simulink model "closed_pi_VS"  (R2015b)
settings: Solver=ode15s  StartTime=0.0  StopTime=16000  MaxStep=10  RelTol=1e-3
values from neighbouring files (symbols this model uses):
  alfa = 3.0    (= 3)    [project_162.m]
  den_VS = [tau_i 0]    [project_162.m]
  M1 = 6000    [project_162.m]
  M10 = 6000    [project_162.m]
  M2 = 50    [project_162.m]
  M3 = 50    [project_162.m]
  M4 = 50    [project_162.m]
  M5 = 50    [project_162.m]
  M6 = 50    [project_162.m]
  M7 = 50    [project_162.m]
  M8 = 50    [project_162.m]
  M9 = 50    [project_162.m]
  num_VS = [kc_VS*tau_i kc_VS]    [project_162.m]
  VS_final = 0    [project_162.m]
  VS_steptime = 0    [project_162.m]
settings Model: Creator=chris  LastModifiedBy=chris
settings DataIOCC: SaveFormat=Array  SignalLoggingSaveFormat=ModelDataLogs
settings OptimizationCC: InitFltsAndDblsToZero=on
settings DebuggingCC: SaveWithParameterizedLinksMsg=none  UnderspecifiedInitializationDetection=Classic  MergeDetectMultiDrivingBlocksExec=none  SignalResolutionControl=TryResolveAllWithWarning  SolverPrmCheckMsg=warning  MultiTaskDSMMsg=warning  MultiTaskCondExecSysMsg=none  FcnCallInpInsideContextMsg=UseLocalSettings
settings HardwareCC: ProdBitPerPointer=32  ProdLargestAtomicFloat=None  ProdIntDivRoundTo=Undefined  ProdEndianess=Unspecified  ProdWordSize=32  ProdHWDeviceType=32-bit Generic
settings GRTTargetCC: TargetFcnLib=ansi_tfl_tmw.mat  CombineOutputUpdateFcns=off  GRTInterface=on
settings ConfigComp: CovModelRefEnable=Off

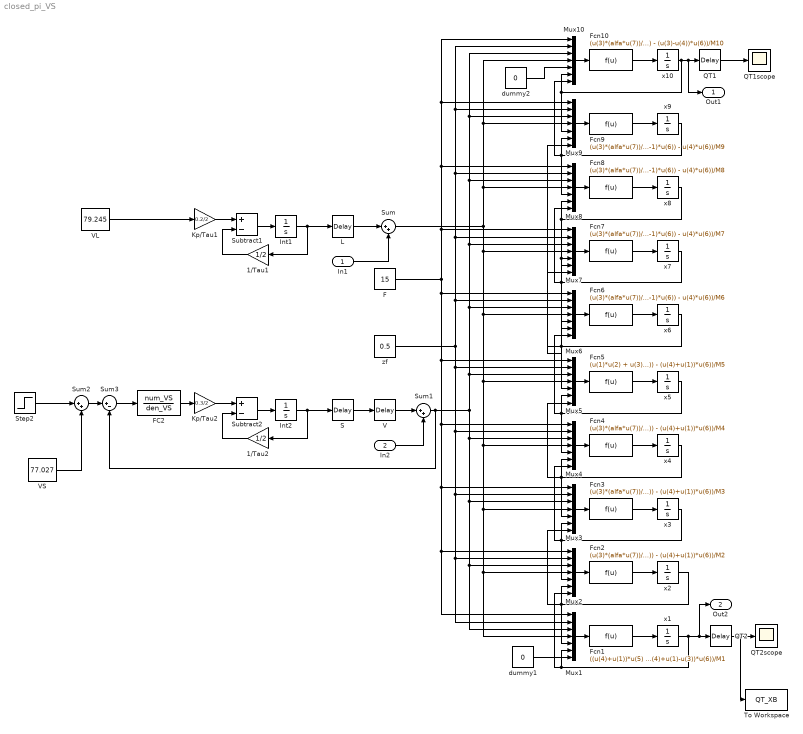
== system closed_pi_VS ==
  In1 : Inport
  In2 : Inport  Port=2
  1/Tau1 : Gain  Gain=1/2
  1/Tau2 : Gain  Gain=1/2
  F : Constant  Value=15
  FC2 : TransferFcn  Numerator=num_VS  Denominator=den_VS
  Fcn1 : Fcn  Expr=((u(4)+u(1))*u(5) - u(3)*(alfa*u(6))/(1+(alfa-1)*u(6)) - (u(4)+u(1)-u(3))*u(6))/M1
  Fcn10 : Fcn  Expr=(u(3)*(alfa*u(7))/(1+(alfa-1)*u(7)) - u(4)*u(6) - (u(3)-u(4))*u(6))/M10
  Fcn2 : Fcn  Expr=(u(3)*(alfa*u(7))/(1+(alfa-1)*u(7)) + (u(4)+u(1))*u(5) - u(3)*(alfa*u(6))/(1+(alfa-1)*u(6)) - (u(4)+u(1))*u(6))/M2
  Fcn3 : Fcn  Expr=(u(3)*(alfa*u(7))/(1+(alfa-1)*u(7)) + (u(4)+u(1))*u(5) - u(3)*(alfa*u(6))/(1+(alfa-1)*u(6)) - (u(4)+u(1))*u(6))/M3
  Fcn4 : Fcn  Expr=(u(3)*(alfa*u(7))/(1+(alfa-1)*u(7)) + (u(4)+u(1))*u(5) - u(3)*(alfa*u(6))/(1+(alfa-1)*u(6)) - (u(4)+u(1))*u(6))/M4
  Fcn5 : Fcn  Expr=(u(1)*u(2) + u(3)*(alfa*u(7))/(1+(alfa-1)*u(7)) + u(4)*u(5) - u(3)*(alfa*u(6))/(1+(alfa-1)*u(6)) - (u(4)+u(1))*u(6))/M5
  Fcn6 : Fcn  Expr=(u(3)*(alfa*u(7))/(1+(alfa-1)*u(7)) + u(4)*u(5) - u(3)*(alfa*u(6))/(1+(alfa-1)*u(6)) - u(4)*u(6))/M6
  Fcn7 : Fcn  Expr=(u(3)*(alfa*u(7))/(1+(alfa-1)*u(7)) + u(4)*u(5) - u(3)*(alfa*u(6))/(1+(alfa-1)*u(6)) - u(4)*u(6))/M7
  Fcn8 : Fcn  Expr=(u(3)*(alfa*u(7))/(1+(alfa-1)*u(7)) + u(4)*u(5) - u(3)*(alfa*u(6))/(1+(alfa-1)*u(6)) - u(4)*u(6))/M8
  Fcn9 : Fcn  Expr=(u(3)*(alfa*u(7))/(1+(alfa-1)*u(7)) + u(4)*u(5) - u(3)*(alfa*u(6))/(1+(alfa-1)*u(6)) - u(4)*u(6))/M9
  Int1 : Integrator  InitialCondition=15.849
  Int2 : Integrator  InitialCondition=23.108
  Kp/Tau1 : Gain  Gain=0.2/2
  Kp/Tau2 : Gain  Gain=0.3/2
  L : TransportDelay  InitialOutput=15.849
  Mux{1..10} (10 alike) : Mux  Inputs=7
  QT1 : TransportDelay  DelayTime=900  InitialOutput=0.980
  QT1scope : Scope
  QT2 : TransportDelay  DelayTime=900  InitialOutput=0.050
  QT2scope : Scope
  S : TransportDelay  InitialOutput=23.108
  Step2 : Step  Time=VS_steptime  After=VS_final  SampleTime=0
  Subtract1 : Sum  Inputs=+-
  Subtract2 : Sum  Inputs=+-
  Sum : Sum  Inputs=|++
  Sum1 : Sum  Inputs=|++
  Sum2 : Sum  Inputs=|++
  Sum3 : Sum  Inputs=|+-
  To Workspace : ToWorkspace  VariableName=QT_XB  SaveFormat=Structure With Time  SampleTime=-1
  V : TransportDelay  DelayTime=30  InitialOutput=23.108
  VL : Constant  Value=79.245
  VS : Constant  Value=77.027
  dummy1 : Constant  Value=0
  dummy2 : Constant  Value=0
  x1 : Integrator  InitialCondition=0.050
  x10 : Integrator  InitialCondition=0.980
  x2 : Integrator  InitialCondition=0.115
  x3 : Integrator  InitialCondition=0.222
  x4 : Integrator  InitialCondition=0.358
  x5 : Integrator  InitialCondition=0.482
  x6 : Integrator  InitialCondition=0.624
  x7 : Integrator  InitialCondition=0.765
  x8 : Integrator  InitialCondition=0.874
  x9 : Integrator  InitialCondition=0.942
  zf : Constant  Value=0.5
  Out1 : Outport
  Out2 : Outport  Port=2
  wires:
  Mux1/1 -> Fcn1/1
  Fcn1/1 -> x1/1
  x1/1 -> Mux1/6, Mux2/7, QT2/1, Out2/1
  Mux2/1 -> Fcn2/1
  Fcn2/1 -> x2/1
  x2/1 -> Mux2/6, Mux1/5, Mux3/7
  Mux3/1 -> Fcn3/1
  Fcn3/1 -> x3/1
  Mux4/1 -> Fcn4/1
  Fcn4/1 -> x4/1
  x4/1 -> Mux3/5, Mux4/6, Mux5/7
  x3/1 -> Mux3/6, Mux2/5, Mux4/7
  Mux5/1 -> Fcn5/1
  Fcn5/1 -> x5/1
  x5/1 -> Mux4/5, Mux5/6, Mux6/7
  Mux6/1 -> Fcn6/1
  Fcn6/1 -> x6/1
  x6/1 -> Mux6/6, Mux5/5, Mux7/7
  Mux7/1 -> Fcn7/1
  Fcn7/1 -> x7/1
  x7/1 -> Mux7/6, Mux6/5, Mux8/7
  Mux8/1 -> Fcn8/1
  Fcn8/1 -> x8/1
  x8/1 -> Mux7/5, Mux9/7, Mux8/6
  Mux9/1 -> Fcn9/1
  Fcn9/1 -> x9/1
  x9/1 -> Mux9/6, Mux8/5, Mux10/7
  Mux10/1 -> Fcn10/1
  Fcn10/1 -> x10/1
  x10/1 -> Mux10/6, Mux9/5, QT1/1, Out1/1
  F/1 -> Mux1/1, Mux2/1, Mux3/1, Mux4/1, Mux5/1, Mux6/1, Mux10/1, Mux9/1, Mux8/1, Mux7/1
  zf/1 -> Mux10/2, Mux9/2, Mux8/2, Mux7/2, Mux6/2, Mux5/2, Mux4/2, Mux3/2, Mux1/2, Mux2/2
  S/1 -> V/1
  QT1/1 -> QT1scope/1
  QT2/1 -> To Workspace/1, QT2scope/1
  Subtract1/1 -> Int1/1
  Int1/1 -> 1/Tau1/1, L/1
  1/Tau1/1 -> Subtract1/2
  Kp/Tau1/1 -> Subtract1/1
  Subtract2/1 -> Int2/1
  Int2/1 -> 1/Tau2/1, S/1
  1/Tau2/1 -> Subtract2/2
  Kp/Tau2/1 -> Subtract2/1
  V/1 -> Sum1/1
  L/1 -> Sum/1
  dummy2/1 -> Mux10/5
  dummy1/1 -> Mux1/7
  Sum/1 -> Mux4/4, Mux3/4, Mux1/4, Mux2/4, Mux5/4, Mux6/4, Mux7/4, Mux10/4, Mux9/4, Mux8/4
  In1/1 -> Sum/2
  Sum1/1 -> Sum3/2, Mux3/3, Mux1/3, Mux2/3, Mux4/3, Mux10/3, Mux9/3, Mux8/3, Mux7/3, Mux6/3, Mux5/3
  In2/1 -> Sum1/2
  VL/1 -> Kp/Tau1/1
  Step2/1 -> Sum2/1
  VS/1 -> Sum2/2
  Sum2/1 -> Sum3/1
  FC2/1 -> Kp/Tau2/1
  Sum3/1 -> FC2/1
